simulink model "bh_linearise_6dof_multiple_PORTS"  (R2016b)
settings: Solver=ode23s  StartTime=0.0  StopTime=20  FixedStep=0.001  RelTol=1e-5  EnableMultiTasking=on
undefined symbols (not defined in the file or in its folder): P_veh
libraries: bh_6dof_LIBRARY x1
settings Model: Creator=bhorton  LastModifiedBy=bhorton
settings DataIOCC: SaveOutput=off  SignalLogging=off  DSMLogging=off  VisualizeSimOutput=off  SaveTime=off
settings OptimizationCC: LifeSpan=inf
settings DebuggingCC: AllowSymbolicDim=off  SFUnexpectedBacktrackingDiag=warning  SFNoUnconditionalDefaultTransitionDiag=warning  SFExecutionAtInitializationDiag=none
settings ModelReferenceCC: PropagateSignalLabelsOutOfModel=off
settings GRTTargetCC: TargetLangStandard=C89/C90 (ANSI)
settings ConfigComp: CovMetricSettings=dw  CovHtmlReporting=on  CovSaveCumulativeToWorkspaceVar=on  CovSaveSingleToWorkspaceVar=on  CovExternalEMLEnable=off

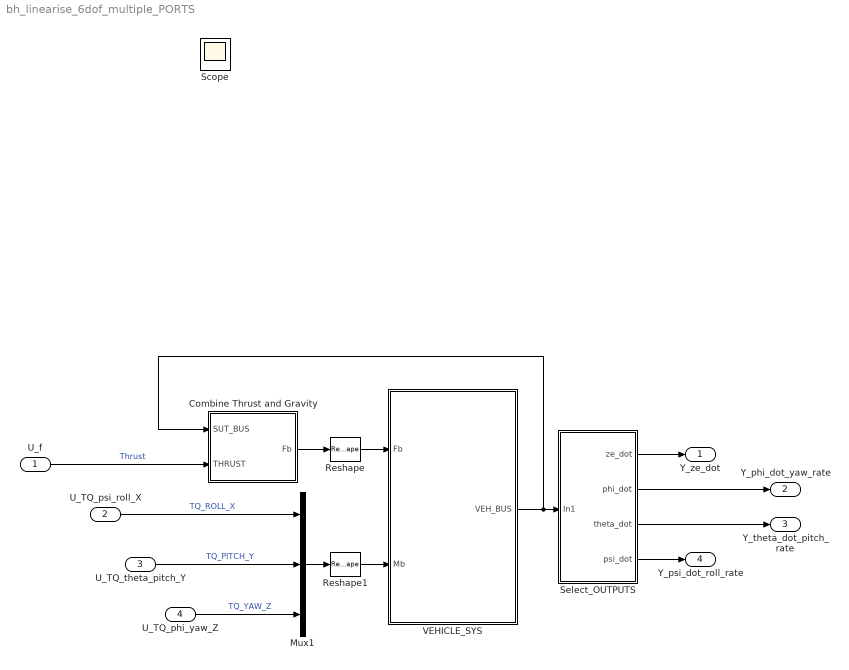
== system bh_linearise_6dof_multiple_PORTS ==
  U_f : Inport
  U_TQ_psi_roll_X : Inport  Port=2
  U_TQ_theta_pitch_Y : Inport  Port=3
  U_TQ_phi_yaw_Z : Inport  Port=4
  Combine Thrust and Gravity : Subsystem
  Mux1 : Mux  Inputs=3
  Reshape : Reshape  OutputDimensionality=Column vector (2-D)
  Reshape1 : Reshape  OutputDimensionality=Column vector (2-D)
  Select_OUTPUTS : Subsystem
  VEHICLE_SYS : Subsystem
  Y_ze_dot : Outport
  Y_phi_dot_yaw_rate : Outport  Port=2
  Y_theta_dot_pitch_rate : Outport  Port=3
  Y_psi_dot_roll_rate : Outport  Port=4
  Scope : Scope
  wires:
  Combine Thrust and Gravity/1(Fb) -> Reshape/1
  Reshape/1 -> VEHICLE_SYS/1(Fb)
  Reshape1/1 -> VEHICLE_SYS/2(Mb)
  Mux1/1 -> Reshape1/1
  U_f/1 -> Combine Thrust and Gravity/2(THRUST)  "Thrust"
  U_TQ_theta_pitch_Y/1 -> Mux1/2  "TQ_PITCH_Y"
  U_TQ_psi_roll_X/1 -> Mux1/1  "TQ_ROLL_X"
  U_TQ_phi_yaw_Z/1 -> Mux1/3  "TQ_YAW_Z"
  VEHICLE_SYS/1(VEH_BUS) -> Combine Thrust and Gravity/1(SUT_BUS), Select_OUTPUTS/1(In1)
  Select_OUTPUTS/1(ze_dot) -> Y_ze_dot/1
  Select_OUTPUTS/2(phi_dot) -> Y_phi_dot_yaw_rate/1
  Select_OUTPUTS/3(theta_dot) -> Y_theta_dot_pitch_rate/1
  Select_OUTPUTS/4(psi_dot) -> Y_psi_dot_roll_rate/1

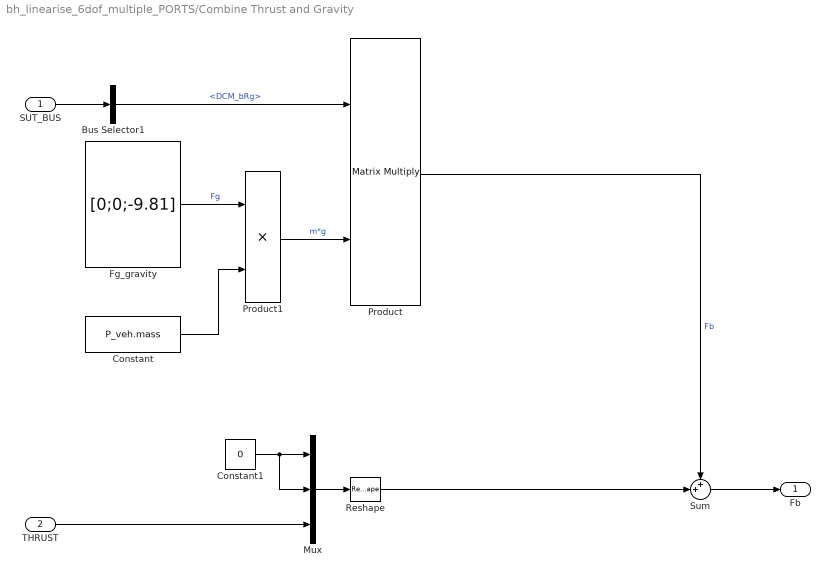
== system bh_linearise_6dof_multiple_PORTS/Combine Thrust and Gravity ==
  SUT_BUS : Inport
  THRUST : Inport  Port=2
  Bus Selector1 : BusSelector  OutputSignals=DCM_bRg
  Constant : Constant  Value=P_veh.mass
  Constant1 : Constant  Value=0
  Fg_gravity : Constant  Value=[0;0;-9.81]  VectorParams1D=off
  Mux : Mux  Inputs=3
  Product : Product  Multiplication=Matrix(*)
  Product1 : Product
  Reshape : Reshape  OutputDimensionality=Column vector (2-D)
  Sum : Sum  Inputs=++|
  Fb : Outport
  wires:
  Sum/1 -> Fb/1
  Constant1/1 -> Mux/2, Mux/1
  THRUST/1 -> Mux/3
  Mux/1 -> Reshape/1
  SUT_BUS/1 -> Bus Selector1/1
  Bus Selector1/1 -> Product/1  "<DCM_bRg>"
  Product1/1 -> Product/2  "m*g"
  Fg_gravity/1 -> Product1/1  "Fg"
  Constant/1 -> Product1/2
  Reshape/1 -> Sum/2
  Product/1 -> Sum/1  "Fb"

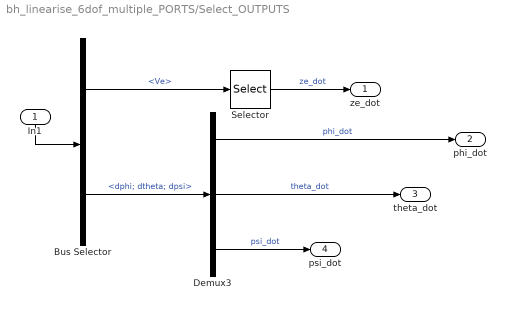
== system bh_linearise_6dof_multiple_PORTS/Select_OUTPUTS ==
  In1 : Inport
  Bus Selector : BusSelector  OutputSignals=Ve,dphi; dtheta; dpsi
  Demux3 : Demux  Outputs=3
  Selector : Selector  InputPortWidth=3  IndexOptions=Index vector (dialog)  Indices=3  OutputSizes=1
  ze_dot : Outport
  phi_dot : Outport  Port=2
  theta_dot : Outport  Port=3
  psi_dot : Outport  Port=4
  wires:
  In1/1 -> Bus Selector/1
  Bus Selector/1 -> Selector/1  "<Ve>"
  Selector/1 -> ze_dot/1  "ze_dot"
  Demux3/3 -> psi_dot/1  "psi_dot"
  Demux3/1 -> phi_dot/1  "phi_dot"
  Demux3/2 -> theta_dot/1  "theta_dot"
  Bus Selector/2 -> Demux3/1  "<dphi; dtheta; dpsi>"

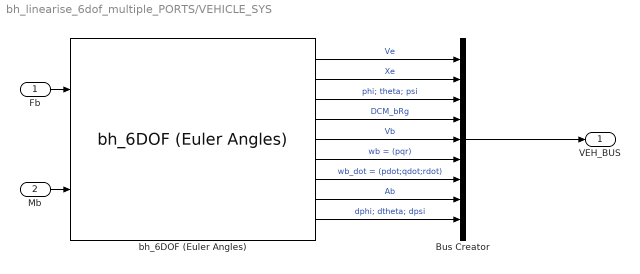
== system bh_linearise_6dof_multiple_PORTS/VEHICLE_SYS ==
  Fb : Inport
  Mb : Inport  Port=2
  Bus Creator : BusCreator  Inputs=9
  bh_6DOF (Euler Angles) : bh_6dof_LIBRARY/MODELS/bh_6DOF (Euler Angles)  inertia_0=P_veh.I  mass_0=P_veh.mass  xme_0=P_veh.Xe_init  Vm_0=P_veh.Vb_init  pm_0=P_veh.wb_init  eul_0=P_veh.eul_init
  VEH_BUS : Outport
  wires:
  Fb/1 -> bh_6DOF (Euler Angles)/1
  Mb/1 -> bh_6DOF (Euler Angles)/2
  bh_6DOF (Euler Angles)/3 -> Bus Creator/3  "phi; theta; psi"
  bh_6DOF (Euler Angles)/2 -> Bus Creator/2  "Xe"
  bh_6DOF (Euler Angles)/1 -> Bus Creator/1  "Ve"
  bh_6DOF (Euler Angles)/4 -> Bus Creator/4  "DCM_bRg"
  bh_6DOF (Euler Angles)/8 -> Bus Creator/8  "Ab"
  bh_6DOF (Euler Angles)/7 -> Bus Creator/7  "wb_dot = (pdot;qdot;rdot)"
  Bus Creator/1 -> VEH_BUS/1
  bh_6DOF (Euler Angles)/5 -> Bus Creator/5  "Vb"
  bh_6DOF (Euler Angles)/6 -> Bus Creator/6  "wb = (pqr)"
  bh_6DOF (Euler Angles)/9 -> Bus Creator/9  "dphi; dtheta; dpsi"
